simulink model "solar_panel"  (R2023b)
settings: Solver=ode14x  StartTime=0.0  StopTime=3*24*3600  FixedStep=1  RelTol=1e-06
PreLoadFcn:
  | sscv_hybrid_solar_panel_data
undefined symbols (not defined in the file): load, panel, pipe
libraries: fl_lib x28, nesl_utility x12, simulink x4, ee_lib x1
CloseFcn:
  | try,close(figHandleSolarInputs),end
  | clear figHandleSolarInputs
  | try,close(figHandlePumpInputs),end
  | clear figHandlePumpInputs
  | try,close(figHandleOptics),end
  | clear figHandleOptics
  | try,close(figHandleOutputs),end
  | clear figHandleOutputs
Description:
  | Photovoltaic Thermal Hybrid Solar Panel.
  | %
settings Model: Creator=The MathWorks, Inc.  LastModifiedBy=Utente PC
settings SolverCC: MaxConsecutiveMinStep=10  AlgebraicLoopSolver=TrustRegion  MaxZcPerStep=1
settings DataIOCC: SaveOutput=off  SignalLogging=off  DSMLogging=off
settings OptimizationCC: ReuseModelBlockBuffer=off
settings DebuggingCC: UnconnectedInputMsg=warning  UnconnectedOutputMsg=warning  UnconnectedLineMsg=warning  ArithmeticOperatorsInVariantConditions=warning
settings ModelReferenceCC: EnableRefExpFcnMdlSchedulingChecks=on
settings SFSimCC: SimUseLocalCustomCode=off
settings RTWCC: RTWUseLocalCustomCode=off  DLArmComputeVersion=19.05
settings SimscapeCC: SimscapeLogType=all  SimscapeLogSimulationStatistics=on  SimscapeLogName=simlog_hybrid_solar_panel  SimscapeLogDataHistory=10000

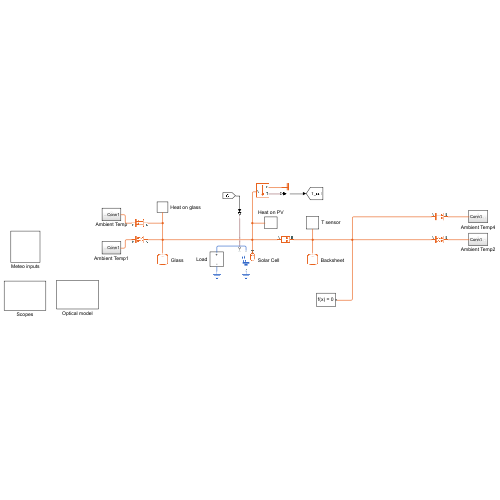
[thumbnail: Simulink's stored preview of the top-level diagram]
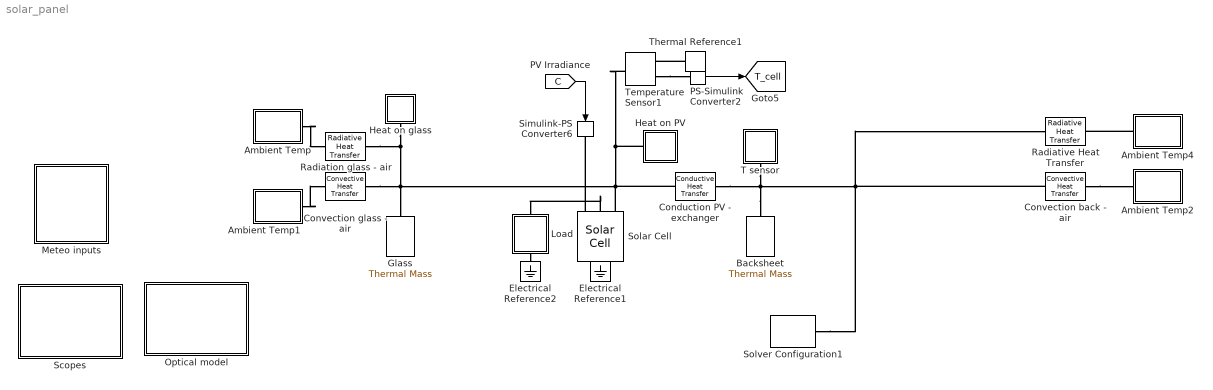
== system solar_panel ==
  Ambient Temp : Subsystem
  Ambient Temp1 : Subsystem
  Ambient Temp2 : Subsystem
  Ambient Temp4 : Subsystem
  Backsheet : fl_lib/Thermal/Thermal Elements/Thermal Mass  mass_type=foundation.enum.constant_variable.constant  mass=panel.heatTransfer.Mbs kg  sp_heat=panel.heatTransfer.Cbs J/kg/K  mass_min=1e-6 kg  num_ports=foundation.enum.numPorts2.one  m_specify=off  m_priority=High  m=1 kg  m_nominal_specify=off  m_nominal_unit=kg  m_nominal_value=1  T_specify=on  T_priority=High  T=panel.initial.Te0 K  T_nominal_specify=off  T_nominal_unit=K  T_nominal_value=1  Q_specify=off  Q_priority=None  Q=0 W  Q_nominal_specify=off  Q_nominal_unit=W  Q_nominal_value=1
  Conduction PV - exchanger : fl_lib/Thermal/Thermal Elements/Conductive Heat Transfer  thermal_type=foundation.enum.ConstantVariableTabulated.Constant  wall_geometry=foundation.enum.ConductionWallGeometry.Planar  area=panel.geometry.Ncell*panel.geometry.Acell m^2  thickness=panel.heatTransfer.Le m  d_in=0.05 m  d_out=0.1 m  L=1 m  th_cond_min=10 W/(K*m)  th_cond=panel.heatTransfer.ke W/(m*K)  th_cond_TLU=[413, 401, 392, 383, 371, 357, 342] W/(K*m)  temp_TLU=[200, 273, 400, 600, 800, 1000, 1200] K  T_specify=off  T_priority=None  T=0 K  T_nominal_specify=off  T_nominal_unit=K  T_nominal_value=1  Q_specify=off  Q_priority=None  Q=0 W  Q_nominal_specify=off  Q_nominal_unit=W  Q_nominal_value=1
  Convection back - air : fl_lib/Thermal/Thermal Elements/Convective Heat Transfer  thermal_type=foundation.enum.constant_variable.constant  area=panel.geometry.Ncell*panel.geometry.Acell m^2  heat_tr_coeff=panel.heatTransfer.hba W/(m^2 * K)  min_heat_tr_coeff=1e-3 W/(K*m^2)  T_specify=off  T_priority=None  T=0 K  T_nominal_specify=off  T_nominal_unit=K  T_nominal_value=1  Q_specify=off  Q_priority=None  Q=0 W  Q_nominal_specify=off  Q_nominal_unit=W  Q_nominal_value=1
  Convection glass - air : fl_lib/Thermal/Thermal Elements/Convective Heat Transfer  thermal_type=foundation.enum.constant_variable.constant  area=panel.geometry.Ncell*panel.geometry.Acell m^2  heat_tr_coeff=panel.heatTransfer.hga W/(m^2 * K)  min_heat_tr_coeff=1e-3 W/(K*m^2)  T_specify=off  T_priority=None  T=0 K  T_nominal_specify=off  T_nominal_unit=K  T_nominal_value=1  Q_specify=off  Q_priority=None  Q=0 W  Q_nominal_specify=off  Q_nominal_unit=W  Q_nominal_value=1
  Electrical Reference1 : fl_lib/Electrical/Electrical Elements/Electrical Reference
  Electrical Reference2 : fl_lib/Electrical/Electrical Elements/Electrical Reference
  Glass : fl_lib/Thermal/Thermal Elements/Thermal Mass  mass_type=foundation.enum.constant_variable.constant  mass=panel.heatTransfer.Mg kg  sp_heat=panel.heatTransfer.Cg J/kg/K  mass_min=1e-6 kg  num_ports=foundation.enum.numPorts2.one  m_specify=off  m_priority=High  m=1 kg  m_nominal_specify=off  m_nominal_unit=kg  m_nominal_value=1  T_specify=on  T_priority=High  T=panel.initial.Tg0 K  T_nominal_specify=off  T_nominal_unit=K  T_nominal_value=1  Q_specify=off  Q_priority=None  Q=0 W  Q_nominal_specify=off  Q_nominal_unit=W  Q_nominal_value=1
  Heat on PV : Subsystem
  Heat on glass : Subsystem
  Load : Subsystem
  Meteo inputs : Subsystem
  Optical model : Subsystem
  PS-Simulink Converter2 : nesl_utility/PS-Simulink Converter  PhysicalDomain=network_engine_domain  SubClassName=ps_output  LeftPortType=input  RightPortType=output  PseudoPeriodic=off  Frequencies=[]  VectorFormat=inherit  Unit=K  AffineConversion=off
  Radiation glass - air : fl_lib/Thermal/Thermal Elements/Radiative Heat Transfer  area=panel.geometry.Ncell*panel.geometry.Acell m^2  rad_tr_coeff=5.670367e-8*panel.heatTransfer.epsg W/(m^2*K^4)  T_specify=off  T_priority=None  T=0 K  T_nominal_specify=off  T_nominal_unit=K  T_nominal_value=1  Q_specify=off  Q_priority=None  Q=0 W  Q_nominal_specify=off  Q_nominal_unit=W  Q_nominal_value=1
      settings: InternalSimscapePortConfiguration="{\"Bottom\":[],\"Left\":[{\"id\":\"A\",\"label\":\"A\",\"type\":\"foundation.thermal.thermal\"}],\"Right\":[{\"id\":\"B\",\"label\":\"B\",\"type\":\"foundation.thermal.thermal\"}],\"Top\":[]}"
  Radiative Heat Transfer : fl_lib/Thermal/Thermal Elements/Radiative Heat Transfer  area=panel.geometry.Ncell*panel.geometry.Acell m^2  rad_tr_coeff=5.670367e-8/(1/pipe.emiss + 1/pipe.emiss_bricks - 1) W/(K^4*m^2)  T_specify=off  T_priority=None  T=0 K  T_nominal_specify=off  T_nominal_unit=K  T_nominal_value=1  Q_specify=off  Q_priority=None  Q=0 W  Q_nominal_specify=off  Q_nominal_unit=W  Q_nominal_value=1
      settings: InternalSimscapePortConfiguration="{\"Bottom\":[],\"Left\":[{\"id\":\"A\",\"label\":\"A\",\"type\":\"foundation.thermal.thermal\"}],\"Right\":[{\"id\":\"B\",\"label\":\"B\",\"type\":\"foundation.thermal.thermal\"}],\"Top\":[]}"
  Scopes : Subsystem
  Simulink-PS Converter6 : nesl_utility/Simulink-PS Converter  PhysicalDomain=network_engine_domain  SubClassName=ps_input  LeftPortType=input  RightPortType=output  PseudoPeriodic=off  Frequencies=[]  NoiseDistribution=none  NoiseParameters=[]  Unit=W/m^2  AffineConversion=off  FilteringAndDerivatives=provide  SimscapeFilterOrder=1  InputFilterTimeConstant=0.001  UdotUserProvided=0
  Solar Cell : ee_lib/Sources/Solar Cell  prm=1  Isc=panel.pv.Isc A  Voc=panel.pv.Voc V  Is=1e-6 A  Is2=0 A  Iph=7.34 A  Ir0=panel.pv.Ir0 W/m^2  ec=panel.pv.ec  N2=2  Rs=panel.pv.Rs Ohm  Rp=inf Ohm  N_series=panel.geometry.Ncell  N_parallel=1  TIPH1=panel.pv.TIPH1 1/K  EG=panel.pv.EG eV  TXIS1=panel.pv.TXIS1  TXIS2=3  TRS1=panel.pv.TRS1  TRP1=0  Tmeas=panel.pv.Tmeas degC  TFIXED=25 degC  thermal_mass=panel.heatTransfer.Mpv*panel.heatTransfer.Cpv J/K  initial_temperature=panel.initial.Tpv0 K
      settings: InternalSimscapePortConfiguration="{\"Bottom\":[],\"Left\":[{\"id\":\"Ir\",\"label\":\"Ir\",\"type\":\"input\"},{\"id\":\"p\",\"label\":\"+\",\"type\":\"foundation.electrical.electrical\"},{\"id\":\"H\",\"label\":\"H\",\"type\":\"foundation.thermal.thermal\"}],\"Right\":[{\"id\":\"n\",\"label\":\"-\",\"type\":\"foundation.electrical.electrical\"}],\"Top\":[]}"
  Solver Configuration1 : nesl_utility/Solver Configuration  PhysicalDomain=network_engine_domain  SubClassName=solver  LeftPortType=input  RightPortType=generic  Tones=[]  Harmonics=[]  SimulateNoise=off  Profile=off  UseLocalSampling=off  EnableSwitchedLinearOptims=on  FrequencyDomain=off  UseCCode=off  RelTol=0.001  AbsTol=0.001  MinStep=1e-09  ToWorkspace=off  RevertToSquareIcSolve=off  NumHomotopyIterations=100  PhasorMode=off  PhasorModeNumHarmonics=1  ConsistencySolver=NEWTON_XTOL_AFTER_FTOL  IndexReductionMethod=DerivativeReplacement  DoDC=off  ResidualTolerance=1e-09  ConsistencyTolSource=GLOBAL  ConsistencyAbsTol=0.001  ConsistencyRelTol=0.001  ConsistencyTolFactor=0.001  UseLocalSolver=off  LocalSolverChoice=NE_BACKWARD_EULER_ADVANCER  ResolveIndetEquations=on  FunctionEvalNumThread=1  LocalSolverSampleTime=0.001  DoFixedCost=off  MaxNonlinIter=3  MaxModeIter=2  ComputeImpulses=off  ImpulseIterations=2  LinearAlgebra=auto  LinearAlgebraNumThread=0  EquationFormulation=NE_TIME_EF  DelaysMemoryBudget=1024  AutomaticFiltering=on  FilteringTimeConstant=0.001  PartitionStorageMethod=AS_NEEDED  PartitionMemoryBudget=1024  PartitionMethod=ROBUST  MultibodyUseLocalSolver=off  MultibodyLocalSolverChoice=ODE1  MultibodyLocalSolverSampleTime=0.001
  T sensor : Subsystem
  Temperature Sensor1 : fl_lib/Thermal/Thermal Sensors/Temperature Sensor  temperature_measure=foundation.enum.MeasurementReference.difference
  Thermal Reference1 : fl_lib/Thermal/Thermal Elements/Thermal Reference
  tag scope: T_cell=global
  wires:
  [C] -> Simulink-PS Converter6/1
  PS-Simulink Converter2/1 -> [T_cell]
  connections:
  Convection glass - air/LConn1 -- Temperature Sensor1/LConn1 -- Heat on PV/LConn1 -- Conduction PV - exchanger/LConn1 -- Solar Cell/LConn3 -- Heat on glass/LConn1 -- Radiation glass - air/LConn1 -- Glass/LConn1
  Solar Cell/LConn1 -- Simulink-PS Converter6/RConn1
  Solar Cell/RConn1 -- Electrical Reference1/LConn1
  Load/LConn1 -- Electrical Reference2/LConn1
  Solar Cell/LConn2 -- Load/RConn1
  Ambient Temp/LConn1 -- Radiation glass - air/RConn1
  Ambient Temp1/LConn1 -- Convection glass - air/RConn1
  Backsheet/LConn1 -- Conduction PV - exchanger/RConn1 -- T sensor/LConn1 -- Solver Configuration1/RConn1 -- Radiative Heat Transfer/LConn1 -- Convection back - air/LConn1
  Convection back - air/RConn1 -- Ambient Temp2/LConn1
  Thermal Reference1/LConn1 -- Temperature Sensor1/RConn1
  Temperature Sensor1/RConn2 -- PS-Simulink Converter2/LConn1
  Ambient Temp4/LConn1 -- Radiative Heat Transfer/RConn1

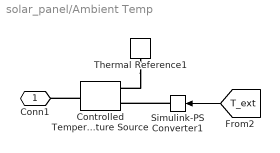
== system solar_panel/Ambient Temp ==
  Controlled Temperature Source : fl_lib/Thermal/Thermal Sources/Controlled Temperature Source
  Simulink-PS Converter1 : nesl_utility/Simulink-PS Converter  PhysicalDomain=network_engine_domain  SubClassName=ps_input  LeftPortType=input  RightPortType=output  PseudoPeriodic=off  Frequencies=[]  NoiseDistribution=none  NoiseParameters=[]  Unit=K  AffineConversion=off  FilteringAndDerivatives=provide  SimscapeFilterOrder=1  InputFilterTimeConstant=0.001  UdotUserProvided=0
  Thermal Reference1 : fl_lib/Thermal/Thermal Elements/Thermal Reference
  Conn1 : PMIOPort  Side=Left
  wires:
  [T_ext] -> Simulink-PS Converter1/1
  connections:
  Simulink-PS Converter1/RConn1 -- Controlled Temperature Source/RConn1
  Thermal Reference1/LConn1 -- Controlled Temperature Source/RConn2
  Controlled Temperature Source/LConn1 -- Conn1/RConn1

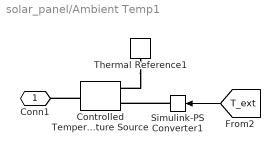
== system solar_panel/Ambient Temp1 ==
  Controlled Temperature Source : fl_lib/Thermal/Thermal Sources/Controlled Temperature Source
  Simulink-PS Converter1 : nesl_utility/Simulink-PS Converter  PhysicalDomain=network_engine_domain  SubClassName=ps_input  LeftPortType=input  RightPortType=output  PseudoPeriodic=off  Frequencies=[]  NoiseDistribution=none  NoiseParameters=[]  Unit=K  AffineConversion=off  FilteringAndDerivatives=provide  SimscapeFilterOrder=1  InputFilterTimeConstant=0.001  UdotUserProvided=0
  Thermal Reference1 : fl_lib/Thermal/Thermal Elements/Thermal Reference
  Conn1 : PMIOPort  Side=Left
  wires:
  [T_ext] -> Simulink-PS Converter1/1
  connections:
  Controlled Temperature Source/LConn1 -- Conn1/RConn1
  Thermal Reference1/LConn1 -- Controlled Temperature Source/RConn2
  Simulink-PS Converter1/RConn1 -- Controlled Temperature Source/RConn1

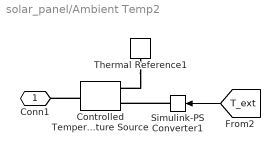
== system solar_panel/Ambient Temp2 ==
  Controlled Temperature Source : fl_lib/Thermal/Thermal Sources/Controlled Temperature Source
  Simulink-PS Converter1 : nesl_utility/Simulink-PS Converter  PhysicalDomain=network_engine_domain  SubClassName=ps_input  LeftPortType=input  RightPortType=output  PseudoPeriodic=off  Frequencies=[]  NoiseDistribution=none  NoiseParameters=[]  Unit=K  AffineConversion=off  FilteringAndDerivatives=provide  SimscapeFilterOrder=1  InputFilterTimeConstant=0.001  UdotUserProvided=0
  Thermal Reference1 : fl_lib/Thermal/Thermal Elements/Thermal Reference
  Conn1 : PMIOPort  Side=Left
  wires:
  [T_ext] -> Simulink-PS Converter1/1
  connections:
  Simulink-PS Converter1/RConn1 -- Controlled Temperature Source/RConn1
  Thermal Reference1/LConn1 -- Controlled Temperature Source/RConn2
  Controlled Temperature Source/LConn1 -- Conn1/RConn1

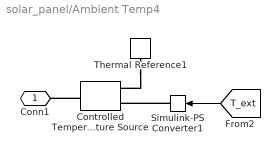
== system solar_panel/Ambient Temp4 ==
  Controlled Temperature Source : fl_lib/Thermal/Thermal Sources/Controlled Temperature Source
  Simulink-PS Converter1 : nesl_utility/Simulink-PS Converter  PhysicalDomain=network_engine_domain  SubClassName=ps_input  LeftPortType=input  RightPortType=output  PseudoPeriodic=off  Frequencies=[]  NoiseDistribution=none  NoiseParameters=[]  Unit=K  AffineConversion=off  FilteringAndDerivatives=provide  SimscapeFilterOrder=1  InputFilterTimeConstant=0.001  UdotUserProvided=0
  Thermal Reference1 : fl_lib/Thermal/Thermal Elements/Thermal Reference
  Conn1 : PMIOPort  Side=Left
  wires:
  [T_ext] -> Simulink-PS Converter1/1
  connections:
  Controlled Temperature Source/LConn1 -- Conn1/RConn1
  Thermal Reference1/LConn1 -- Controlled Temperature Source/RConn2
  Simulink-PS Converter1/RConn1 -- Controlled Temperature Source/RConn1

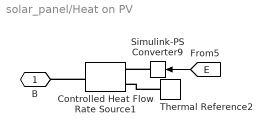
== system solar_panel/Heat on PV ==
  Controlled Heat Flow Rate Source1 : fl_lib/Thermal/Thermal Sources/Controlled Heat Flow Rate Source
  Simulink-PS Converter9 : nesl_utility/Simulink-PS Converter  PhysicalDomain=network_engine_domain  SubClassName=ps_input  LeftPortType=input  RightPortType=output  PseudoPeriodic=off  Frequencies=[]  NoiseDistribution=none  NoiseParameters=[]  Unit=W  AffineConversion=off  FilteringAndDerivatives=provide  SimscapeFilterOrder=1  InputFilterTimeConstant=0.001  UdotUserProvided=0
  Thermal Reference2 : fl_lib/Thermal/Thermal Elements/Thermal Reference
  B : PMIOPort  Side=Left
  wires:
  [E] -> Simulink-PS Converter9/1
  connections:
  Simulink-PS Converter9/RConn1 -- Controlled Heat Flow Rate Source1/RConn1
  Thermal Reference2/LConn1 -- Controlled Heat Flow Rate Source1/RConn2
  Controlled Heat Flow Rate Source1/LConn1 -- B/RConn1

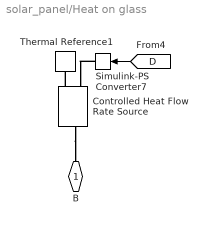
== system solar_panel/Heat on glass ==
  Controlled Heat Flow Rate Source : fl_lib/Thermal/Thermal Sources/Controlled Heat Flow Rate Source
  Simulink-PS Converter7 : nesl_utility/Simulink-PS Converter  PhysicalDomain=network_engine_domain  SubClassName=ps_input  LeftPortType=input  RightPortType=output  PseudoPeriodic=off  Frequencies=[]  NoiseDistribution=none  NoiseParameters=[]  Unit=W  AffineConversion=off  FilteringAndDerivatives=provide  SimscapeFilterOrder=1  InputFilterTimeConstant=0.001  UdotUserProvided=0
  Thermal Reference1 : fl_lib/Thermal/Thermal Elements/Thermal Reference
  B : PMIOPort  Side=Left
  wires:
  [D] -> Simulink-PS Converter7/1
  connections:
  Simulink-PS Converter7/RConn1 -- Controlled Heat Flow Rate Source/RConn1
  Controlled Heat Flow Rate Source/RConn2 -- Thermal Reference1/LConn1
  Controlled Heat Flow Rate Source/LConn1 -- B/RConn1

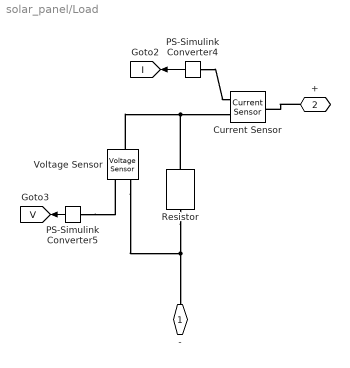
== system solar_panel/Load ==
  Current Sensor : fl_lib/Electrical/Electrical Sensors/Current Sensor
  PS-Simulink Converter4 : nesl_utility/PS-Simulink Converter  PhysicalDomain=network_engine_domain  SubClassName=ps_output  LeftPortType=input  RightPortType=output  PseudoPeriodic=off  Frequencies=[]  VectorFormat=1-D array  Unit=1  AffineConversion=off
  PS-Simulink Converter5 : nesl_utility/PS-Simulink Converter  PhysicalDomain=network_engine_domain  SubClassName=ps_output  LeftPortType=input  RightPortType=output  PseudoPeriodic=off  Frequencies=[]  VectorFormat=1-D array  Unit=1  AffineConversion=off
  Resistor : fl_lib/Electrical/Electrical Elements/Resistor  R=load.R Ohm  i_specify=off  i_priority=None  i=0 A  i_nominal_specify=off  i_nominal_unit=A  i_nominal_value=1  v_specify=off  v_priority=None  v=0 V  v_nominal_specify=off  v_nominal_unit=V  v_nominal_value=1
  Voltage Sensor : fl_lib/Electrical/Electrical Sensors/Voltage Sensor
  - : PMIOPort  Side=Left
  + : PMIOPort  Port=2  Side=Right
  tag scope: I=global, V=global
  wires:
  PS-Simulink Converter4/1 -> [I]
  PS-Simulink Converter5/1 -> [V]
  connections:
  +/RConn1 -- Current Sensor/LConn1
  PS-Simulink Converter5/LConn1 -- Voltage Sensor/RConn1
  PS-Simulink Converter4/LConn1 -- Current Sensor/RConn1
  Voltage Sensor/LConn1 -- Resistor/LConn1 -- Current Sensor/RConn2
  Resistor/RConn1 -- Voltage Sensor/RConn2 -- -/RConn1

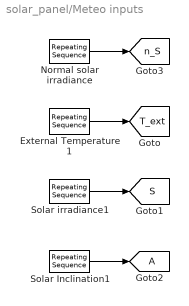
== system solar_panel/Meteo inputs ==
  " Solar Inclination1" : simulink/Sources/Repeating Sequence  rep_seq_t=time  rep_seq_y=inclination
  External Temperature1 : simulink/Sources/Repeating Sequence  rep_seq_t=time  rep_seq_y=t_ext
  Goto2 : Goto  TagVisibility=global
  Normal solar irradiance : simulink/Sources/Repeating Sequence  rep_seq_t=time  rep_seq_y=irradiance_si
  Solar irradiance1 : simulink/Sources/Repeating Sequence  rep_seq_t=time  rep_seq_y=irradiance_ts
  tag scope: S=global, T_ext=global, n_S=global
  wires:
  External Temperature1/1 -> [T_ext]
  " Solar Inclination1"/1 -> Goto2/1
  Solar irradiance1/1 -> [S]
  Normal solar irradiance/1 -> [n_S]

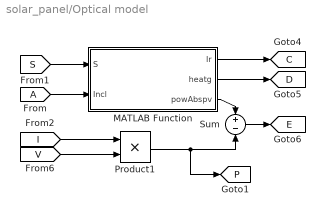
== system solar_panel/Optical model ==
  From : From  TagVisibility=global
  MATLAB Function : MATLAB Function  TreatAsAtomicUnit=on
  Product1 : Product
  Sum : Sum  Inputs=+-
  tag scope: C=global, D=global, E=global, P=global
  wires:
  MATLAB Function/1(Ir) -> [C]
  Sum/1 -> [E]
  MATLAB Function/2(heatg) -> [D]
  MATLAB Function/3(powAbspv) -> Sum/1
  Product1/1 -> Sum/2, [P]
  [I] -> Product1/1
  [V] -> Product1/2
  From/1 -> MATLAB Function/2(Incl)
  [S] -> MATLAB Function/1(S)

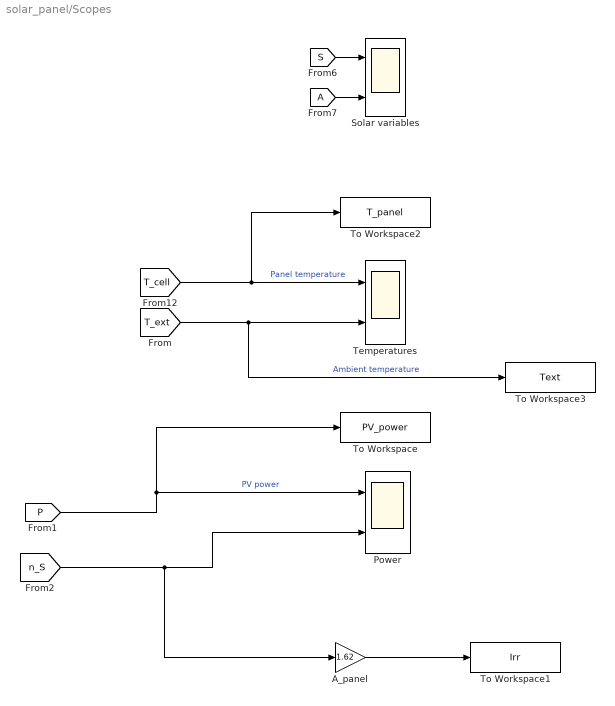
== system solar_panel/Scopes ==
  A_panel : Gain  Gain=1.62
  From7 : From  TagVisibility=global
  Power : Scope  NumInputPorts=2
  Solar variables : Scope  NumInputPorts=2
  Temperatures : Scope  NumInputPorts=2
  To Workspace : ToWorkspace  VariableName=PV_power  SaveFormat=Structure With Time  SampleTime=-1
  To Workspace1 : ToWorkspace  VariableName=Irr  SaveFormat=Structure With Time  SampleTime=-1
  To Workspace2 : ToWorkspace  VariableName=T_panel  SaveFormat=Structure With Time  SampleTime=-1
  To Workspace3 : ToWorkspace  VariableName=Text  SaveFormat=Structure With Time  SampleTime=-1
  wires:
  [P] -> To Workspace/1, Power/1  "PV power"
  [S] -> Solar variables/1
  From7/1 -> Solar variables/2
  [T_ext] -> To Workspace3/1, Temperatures/2  "Ambient temperature"
  [T_cell] -> To Workspace2/1, Temperatures/1  "Panel temperature"
  [n_S] -> A_panel/1, Power/2
  A_panel/1 -> To Workspace1/1

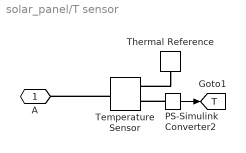
== system solar_panel/T sensor ==
  PS-Simulink Converter2 : nesl_utility/PS-Simulink Converter  PhysicalDomain=network_engine_domain  SubClassName=ps_output  LeftPortType=input  RightPortType=output  PseudoPeriodic=off  Frequencies=[]  VectorFormat=1-D array  Unit=K  AffineConversion=off
  Temperature Sensor : fl_lib/Thermal/Thermal Sensors/Temperature Sensor  temperature_measure=foundation.enum.MeasurementReference.difference
  Thermal Reference : fl_lib/Thermal/Thermal Elements/Thermal Reference
  A : PMIOPort  Side=Left
  tag scope: T=global
  wires:
  PS-Simulink Converter2/1 -> [T]
  connections:
  Temperature Sensor/LConn1 -- A/RConn1
  Thermal Reference/LConn1 -- Temperature Sensor/RConn1
  PS-Simulink Converter2/LConn1 -- Temperature Sensor/RConn2

== matlab function solar_panel/Optical model/MATLAB Function ==
  data: S input; Ir output; Incl input; heatg output; powAbspv output; panel parameter
function [Ir, heatg, powAbspv] = optics(S, Incl, panel)
    
    %This function computes the reflection, absorption and transmission in
    %the glass to compute the irradiation to the PV cells, the heat absorbed 
    %in the glass and the radiation power absorbed in the PV cells,
    %it is based on Fresnel's laws, depending on the incident angle
    
    Ncell = panel.geometry.Ncell;
    Acell = panel.geometry.Acell;
    ng = panel.optical.ng;
    absg = panel.optical.absg;
    dg = panel.optical.dg;
    rpv = panel.optical.rpv;
   

    % Fresnel equations 1st boundary
    r1p =  ( ng^2*cos(Incl) - sqrt(ng^2 - sin(Incl)^2) )^2/( ng^2*cos(Incl) + sqrt( ng^2 - sin(Incl)^2 ) )^2; %P polarization
    r1s =  ( cos(Incl) - sqrt(ng^2 - sin(Incl)^2) )^2/( cos(Incl) + sqrt( ng^2 - sin(Incl)^2 ) )^2; %S polarization
    r1 = 0.5*(r1p + r1s); %Effective reflectance
    t1 = 1-r1;

    nga = 1/ng; %refractive index glass -> air
    th2 = asin(sin(Incl)/ng);  %Snell's law to compute angle of incidence on 2nd boundary

    % Fresnel equations 2nd boundary
    r2p = ( nga^2*cos(th2) - sqrt(nga^2 - sin(th2)^2) )^2/( nga^2*cos(th2) + sqrt( nga^2 - sin(th2)^2 ) )^2 ;
    r2s = ( cos(th2) - sqrt(nga^2 - sin(th2)^2) )^2/( cos(th2) + sqrt( nga^2 - sin(th2)^2 ) )^2 ;
    r2 = 0.5*(r2p + r2s); %Effective reflectance
    t2 = 1 - r2;

    taug = exp(-absg*dg/cos(th2)); 
    
    %Total coefficients for infinite reflections between 2 parallel boundaries
    Transg = t1*taug*t2/(1 - r1*r2*taug^2);
    Reflg = r1 + (t1^2*taug^2*r2)/(1 - r1*r2*taug^2);
    Absg = 1 - Transg - Reflg; 

    Ir = S*Transg; %Irradiation to the PV cells
    heatg = Acell*Ncell*Absg*S; %heat absorbed in the glass
    powAbspv = Acell*Ncell*Transg*(1-rpv)*S; %radiation power absorbed by PV cells. Part of it transforms in electrical power
    
end
